simulink model "model_hippocampus"  (R2019b)
settings: Solver=ode23t  StartTime=0.0  StopTime=30  RelTol=1e-3
values from neighbouring files (symbols this model uses):
  C_T = 0.0000363    (= 3.63e-05)    [calculate_w_from_f_m.m]    (also in create_model-mummel-PC.m; create_model.m)
  D_l = -diag([X_u_u Y_v_v Z_w_w K_p_p M_q_q N_r_r])    [create_model-mummel-PC.m]    (also in create_model.m)
  D_r = -diag([X_u_u Y_v_v Z_w_w K_p_p M_q_q N_r_r])    [create_model-mummel-PC.m]    (also in create_model.m)
  F_to_xrpy = [1 1 1 1;k_m -k_m k_m -k_m ; -h/2 -h/2 h/2 h/2 ; h/2 -h/2 -h/2 h/2]    [calculate_w_from_f_m.m]    (also in create_model-mummel-PC.m = [1 1 1 1;-k_m k_m -k_m k_m ; -h/2 -h/2 h/2 h/2 ; h/2 -h/2 -h; create_model.m = [1 1 1 1;-k_m k_m -k_m k_m ; -h/2 -h/2 h/2 h/2 ; h/2 -h/2 -h)
  K = zeros(4,8)    [create_model-mummel-PC.m]    (also in create_model.m)
  K_list = [0.128176187695 -9.36648609631e-17 -5.00574293925e-18 -3.63491573314e-18 6.34309710249e-16 0.643960726702 1.98403777758e-15 -1.22713415344e-15 -1.03838985673e-16 -1.23229867768e-16 0.996702799245 2.36443760318e-16 ... (16384 elements, 4x8x512)]    [K_list_lqr_1_to_1.mat]    (also in K_list_lqr_moment.mat = [0.215933633332 5.36387970648e-15 5.12418514573e-17 4.256952; K_list_states_to_motor_force.mat = [0.101981554229 0.101981554229 0.101981554229 0.101981554229; create_model-mummel-PC.m = zeros(4,8,N*N*N); create_model.m = zeros(4,8,N*N*N))
  m = 1.47    [create_model-mummel-PC.m]    (also in create_model.m)
  M_A_11 = M_A(1:3,1:3)    [create_model-mummel-PC.m]    (also in create_model.m)
  M_A_22 = M_A(4:6,4:6)    [create_model-mummel-PC.m]    (also in create_model.m)
  M_RB_22 = M_RB(4:6,4:6)    [create_model-mummel-PC.m]    (also in create_model.m)
  M_RB_M_A_INV = inv(M_RB+M_A)    [create_model-mummel-PC.m]    (also in create_model.m)
  mix_matrix_trpy_to_velocity_motor = [[1 1 1 1]' [-1 1 -1 1]' [-1 -1 1 1]' [1 -1 -1 1]']*0.4    [check_correct_index.m]    (also in create_model-mummel-PC.m = [[1 1 1 1]' [-1 1 -1 1]' [-1 -1 1 1]' [1 -1 -1 1]']; create_model.m = [[1 1 1 1]' [-1 1 -1 1]' [-1 -1 1 1]' [1 -1 -1 1]'])
undefined symbols (not defined in the file or in its folder): sigbuilder_block
settings Model: Creator=mummel  LastModifiedBy=tim
settings SolverCC: ZeroCrossAlgorithm=Adaptive
settings DebuggingCC: IgnoredZcDiagnostic=none

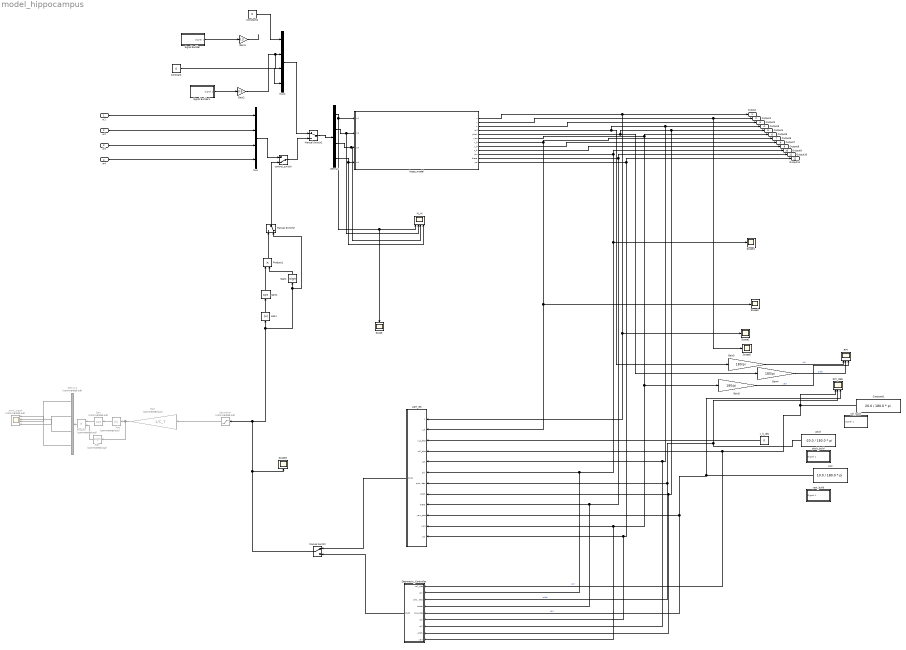
== system model_hippocampus ==
  w1 : Inport
  w2 : Inport  Port=2
  w3 : Inport  Port=3
  w4 : Inport  Port=4
  Abs : Abs  Commented=on
  Abs1 : Abs
  Constant : Constant  Value=0
  Constant1 : Constant  Value=20.0 / 180.0 * pi
  Constant2 : Constant  Value=0
  Demux : Demux
  Demux1 : Demux  Commented=on
  Gain : Gain  Commented=on  Gain=1/C_T
  Gain1 : Gain  Gain=0.3
  Gain2 : Gain  Gain=0.6
  Gain3 : Gain  Gain=180/pi
  Gain4 : Gain  Gain=180/pi
  Gain5 : Gain  Gain=180/pi
  Geometric_Controller : Subsystem
  LQR_GS : Subsystem
  M_IN : Scope  NumInputPorts=4
  Manual Switch : ManualSwitch
  Manual Switch1 : ManualSwitch
  Manual Switch2 : ManualSwitch  CurrentSetting=0
  Mux : Mux
  Mux2 : Mux
  Product : Product  Commented=on
  Product1 : Product
  RPY : Scope  NumInputPorts=3
  RPY_DES : Scope  NumInputPorts=3
  Saturation : Saturate  Commented=on  UpperLimit=7  LowerLimit=-7
  Scope{,1..5} (6 alike) : Scope
  Sign : Signum  Commented=on
  Sign1 : Signum
  Signal Builder : Subsystem  Tag=STV Subsys  LoadFcn=sigbuilder_block('load');  StartFcn=sigbuilder_block('start');  StopFcn=sigbuilder_block('stop');  ClipboardFcn=sigbuilder_block('clipboard');  mask(Sigbuilder block){tuvar=[0:10]}
      mask help: Simulink:masks:SigbuilderBlock_MD
      mask init:
      | if ~strcmp(get_param(bdroot(gcbh),'SimulationStatus'),'stopped') tuvar = sigbuilder_block('maskInit'); end
      settings: CopyFcn=sigbuilder_block('copy');  DeleteFcn=sigbuilder_block('delete');  ModelCloseFcn=sigbuilder_block('modelClose');  PreSaveFcn=sigbuilder_block('preSave');  PauseFcn=sigbuilder_block('pause');  ContinueFcn=sigbuilder_block('continue');  NameChangeFcn=sigbuilder_block('namechange');  OpenFcn=sigbuilder_block('open',[864 302.4 573.726 359.242 ]);  CloseFcn=sigbuilder_block('close');
      mask Display: plot(0, 0, 100, 100,[2, 2, 32, 32, 2], [68, 8, 8, 68, 68],[32, 2], [38, 38], [32, 19, 2],[53, 60, 44], [32, 17, 17, 2],[16, 16, 31, 31]);txt = getActiveGroup(gcbh);text(2, 100, txt,'verticalAlignment', 'top');
  Signal Builder1 : Subsystem  Tag=STV Subsys  LoadFcn=sigbuilder_block('load');  StartFcn=sigbuilder_block('start');  StopFcn=sigbuilder_block('stop');  ClipboardFcn=sigbuilder_block('clipboard');  mask(Sigbuilder block){tuvar=[0:10]}
      mask help: Simulink:masks:SigbuilderBlock_MD
      mask init:
      | if ~strcmp(get_param(bdroot(gcbh),'SimulationStatus'),'stopped') tuvar = sigbuilder_block('maskInit'); end
      settings: CopyFcn=sigbuilder_block('copy');  DeleteFcn=sigbuilder_block('delete');  ModelCloseFcn=sigbuilder_block('modelClose');  PreSaveFcn=sigbuilder_block('preSave');  PauseFcn=sigbuilder_block('pause');  ContinueFcn=sigbuilder_block('continue');  NameChangeFcn=sigbuilder_block('namechange');  OpenFcn=sigbuilder_block('open',[780.75 95.25 558.75 317.25 ]);  CloseFcn=sigbuilder_block('close');
      mask Display: plot(0, 0, 100, 100,[2, 2, 32, 32, 2], [68, 8, 8, 68, 68],[32, 2], [38, 38], [32, 19, 2],[53, 60, 44], [32, 17, 17, 2],[16, 16, 31, 31]);txt = getActiveGroup(gcbh);text(2, 100, txt,'verticalAlignment', 'top');
  Sqrt : Sqrt  Commented=on  SaturateOnIntegerOverflow=on
  Sqrt1 : Sqrt  SaturateOnIntegerOverflow=on
  control_switch : ManualSwitch  CurrentSetting=0
  hippo_model : Subsystem
  pitch : Constant  Value=-20.0 / 180.0 * pi
  pitch_build : Subsystem  Tag=STV Subsys  LoadFcn=sigbuilder_block('load');  StartFcn=sigbuilder_block('start');  StopFcn=sigbuilder_block('stop');  ClipboardFcn=sigbuilder_block('clipboard');  mask(Sigbuilder block){tuvar=[0:10]}
      mask help: Simulink:masks:SigbuilderBlock_MD
      mask init:
      | if ~strcmp(get_param(bdroot(gcbh),'SimulationStatus'),'stopped') tuvar = sigbuilder_block('maskInit'); end
      settings: CopyFcn=sigbuilder_block('copy');  DeleteFcn=sigbuilder_block('delete');  ModelCloseFcn=sigbuilder_block('modelClose');  PreSaveFcn=sigbuilder_block('preSave');  PauseFcn=sigbuilder_block('pause');  ContinueFcn=sigbuilder_block('continue');  NameChangeFcn=sigbuilder_block('namechange');  OpenFcn=sigbuilder_block('open',[437.6 199.2 550.4 400 ]);  CloseFcn=sigbuilder_block('close');
      mask Display: plot(0, 0, 100, 100,[2, 2, 32, 32, 2], [68, 8, 8, 68, 68],[32, 2], [38, 38], [32, 19, 2],[53, 60, 44], [32, 17, 17, 2],[16, 16, 31, 31]);txt = getActiveGroup(gcbh);text(2, 100, txt,'verticalAlignment', 'top');
  pwm_signal : Scope  Commented=on  NumInputPorts=4
  roll_build : Subsystem  Tag=STV Subsys  LoadFcn=sigbuilder_block('load');  StartFcn=sigbuilder_block('start');  StopFcn=sigbuilder_block('stop');  ClipboardFcn=sigbuilder_block('clipboard');  mask(Sigbuilder block){tuvar=[0:10]}
      mask help: Simulink:masks:SigbuilderBlock_MD
      mask init:
      | if ~strcmp(get_param(bdroot(gcbh),'SimulationStatus'),'stopped') tuvar = sigbuilder_block('maskInit'); end
      settings: CopyFcn=sigbuilder_block('copy');  DeleteFcn=sigbuilder_block('delete');  ModelCloseFcn=sigbuilder_block('modelClose');  PreSaveFcn=sigbuilder_block('preSave');  PauseFcn=sigbuilder_block('pause');  ContinueFcn=sigbuilder_block('continue');  NameChangeFcn=sigbuilder_block('namechange');  OpenFcn=sigbuilder_block('open',[437.6 199.2 550.4 400 ]);  CloseFcn=sigbuilder_block('close');
      mask Display: plot(0, 0, 100, 100,[2, 2, 32, 32, 2], [68, 8, 8, 68, 68],[32, 2], [38, 38], [32, 19, 2],[53, 60, 44], [32, 17, 17, 2],[16, 16, 31, 31]);txt = getActiveGroup(gcbh);text(2, 100, txt,'verticalAlignment', 'top');
  x_b_des : Constant  Value=0
  yaw : Constant  Value=10.0 / 180.0 * pi
  yaw_build : Subsystem  Tag=STV Subsys  LoadFcn=sigbuilder_block('load');  StartFcn=sigbuilder_block('start');  StopFcn=sigbuilder_block('stop');  ClipboardFcn=sigbuilder_block('clipboard');  mask(Sigbuilder block){tuvar=[0:10]}
      mask help: Simulink:masks:SigbuilderBlock_MD
      mask init:
      | if ~strcmp(get_param(bdroot(gcbh),'SimulationStatus'),'stopped') tuvar = sigbuilder_block('maskInit'); end
      settings: CopyFcn=sigbuilder_block('copy');  DeleteFcn=sigbuilder_block('delete');  ModelCloseFcn=sigbuilder_block('modelClose');  PreSaveFcn=sigbuilder_block('preSave');  PauseFcn=sigbuilder_block('pause');  ContinueFcn=sigbuilder_block('continue');  NameChangeFcn=sigbuilder_block('namechange');  OpenFcn=sigbuilder_block('open',[437.6 199.2 550.4 400 ]);  CloseFcn=sigbuilder_block('close');
      mask Display: plot(0, 0, 100, 100,[2, 2, 32, 32, 2], [68, 8, 8, 68, 68],[32, 2], [38, 38], [32, 19, 2],[53, 60, 44], [32, 17, 17, 2],[16, 16, 31, 31]);txt = getActiveGroup(gcbh);text(2, 100, txt,'verticalAlignment', 'top');
  Output : Outport
  Output1 : Outport  Port=2
  Output2 : Outport  Port=3
  Output3 : Outport  Port=4
  Output4 : Outport  Port=5
  Output5 : Outport  Port=6
  Output6 : Outport  Port=7
  Output7 : Outport  Port=8
  Output8 : Outport  Port=9
  Output9 : Outport  Port=10
  Output10 : Outport  Port=11
  Output11 : Outport  Port=12
  wires:
  w4/1 -> Mux/4
  w3/1 -> Mux/3
  w2/1 -> Mux/2
  w1/1 -> Mux/1
  hippo_model/1(x) -> Output/1, LQR_GS/1(x), Scope1/1
  hippo_model/2(y) -> Scope5/1, Output1/1
  hippo_model/3(z) -> Output2/1
  hippo_model/4(roll) -> Geometric_Controller/7(roll), LQR_GS/5(roll), Output3/1, Gain3/1
  hippo_model/5(pitch) -> Geometric_Controller/8(pitch), LQR_GS/8(pitch), Output4/1, Gain4/1
  hippo_model/6(yaw) -> Gain5/1, Geometric_Controller/9(yaw), LQR_GS/11(yaw), Output5/1
  hippo_model/7(x_b) -> Output6/1, Scope2/1, LQR_GS/2(x_b)
  hippo_model/8(y_b) -> Output7/1
  hippo_model/9(z_b) -> Output8/1
  hippo_model/10(phi) -> Output9/1, Geometric_Controller/2(phi), LQR_GS/6(phi), Scope4/1
  hippo_model/11(theta) -> Output10/1, LQR_GS/9(theta), Geometric_Controller/4(theta)
  hippo_model/12(psi) -> Output11/1, Geometric_Controller/6(psi), LQR_GS/12(psi)
  Mux/1 -> control_switch/1
  control_switch/1 -> Manual Switch1/2
  Manual Switch/1 -> Scope3/1, Manual Switch2/2, Sign1/1, Abs1/1, Saturation/1
  yaw/1 -> Geometric_Controller/5(yaw_des), LQR_GS/10(yaw_des), RPY_DES/3  "yaw"
  Mux2/1 -> Manual Switch1/1
  Manual Switch1/1 -> Demux/1
  Demux/1 -> hippo_model/1(w1), Scope/1, M_IN/1
  Demux/2 -> hippo_model/2(w2), M_IN/2
  Demux/3 -> hippo_model/3(w3), M_IN/3
  Demux/4 -> hippo_model/4(w4), M_IN/4
  Signal Builder/1(Signal 1) -> Gain1/1
  Geometric_Controller/1(Out1) -> Manual Switch/2
  x_b_des/1 -> LQR_GS/3(x_b_des)
  LQR_GS/1(Out1) -> Manual Switch/1
  Abs/1 -> Sqrt/1
  Sqrt/1 -> Product/1
  Demux1/4 -> pwm_signal/1
  Demux1/3 -> pwm_signal/2
  Demux1/2 -> pwm_signal/4
  Demux1/1 -> pwm_signal/3
  Saturation/1 -> Gain/1
  Gain/1 -> Sign/1, Abs/1
  Sign/1 -> Product/2
  Product/1 -> Demux1/1
  Signal Builder1/1(Signal 1) -> Gain2/1
  Constant1/1 -> RPY_DES/1, Geometric_Controller/1(roll_des), LQR_GS/4(roll_des)  "roll"
  pitch/1 -> Geometric_Controller/3(pitch_des), LQR_GS/7(pitch_des), RPY_DES/2  "pitch"
  Constant/1 -> Mux2/4
  Gain3/1 -> RPY/1  "roll"
  Gain5/1 -> RPY/3  "yaw"
  Gain4/1 -> RPY/2  "pitch"
  Manual Switch2/1 -> control_switch/2
  Abs1/1 -> Sqrt1/1
  Sign1/1 -> Product1/2
  Sqrt1/1 -> Product1/1
  Product1/1 -> Manual Switch2/1
  Gain2/1 -> Mux2/3, Mux2/2
  Gain1/1 -> ?
  Constant2/1 -> Mux2/1

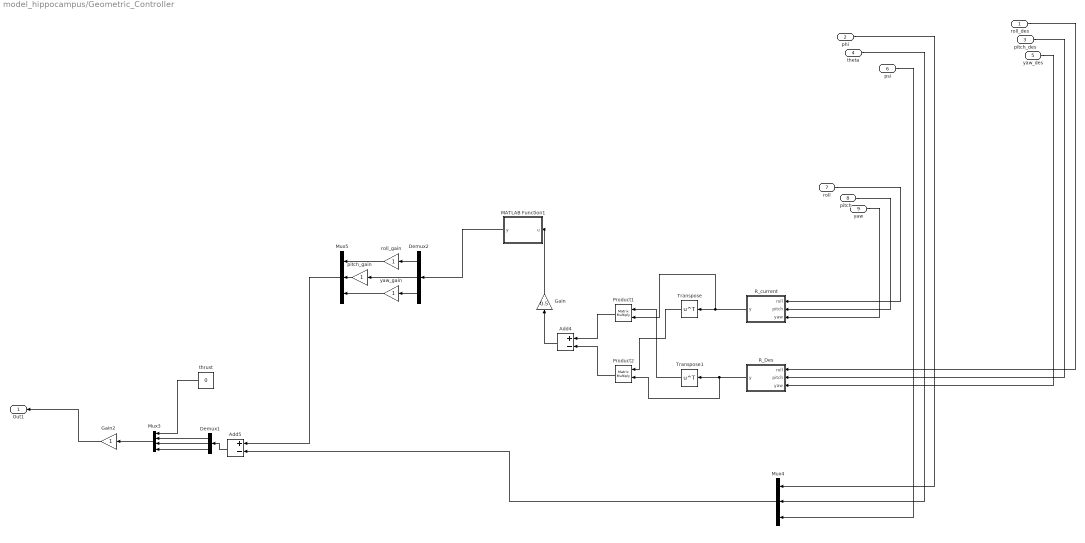
== system model_hippocampus/Geometric_Controller ==
  roll_des : Inport
  phi : Inport  Port=2
  pitch_des : Inport  Port=3
  theta : Inport  Port=4
  yaw_des : Inport  Port=5
  psi : Inport  Port=6
  roll : Inport  Port=7
  pitch : Inport  Port=8
  yaw : Inport  Port=9
  Add4 : Sum  Inputs=+-
  Add5 : Sum  Inputs=+-
  Demux1 : Demux  Outputs=3
  Demux2 : Demux  Outputs=3
  Gain : Gain  Gain=0.5
  Gain2 : Gain
  MATLAB Function1 : MATLAB Function  TreatAsAtomicUnit=on
  Mux3 : Mux
  Mux4 : Mux  Inputs=3
  Mux5 : Mux  Inputs=3
  Product1 : Product  Multiplication=Matrix(*)
  Product2 : Product  Multiplication=Matrix(*)
  R_Des : MATLAB Function  TreatAsAtomicUnit=on
  R_current : MATLAB Function  TreatAsAtomicUnit=on
  Transpose : Math  Operator=transpose  SignedPower=off  SaturateOnIntegerOverflow=on
  Transpose1 : Math  Operator=transpose  SignedPower=off  SaturateOnIntegerOverflow=on
  pitch_gain : Gain
  roll_gain : Gain
  thrust : Constant  Value=0
  yaw_gain : Gain
  Out1 : Outport
  wires:
  Transpose/1 -> Product2/1
  roll_des/1 -> R_Des/1(roll)
  Add5/1 -> Demux1/1
  roll_gain/1 -> Mux5/1
  Demux2/1 -> roll_gain/1
  phi/1 -> Mux4/1
  MATLAB Function1/1(y) -> Demux2/1
  Demux1/3 -> Mux3/4
  Demux1/2 -> Mux3/3
  psi/1 -> Mux4/3
  R_Des/1(y) -> Product2/2, Transpose1/1
  Product2/1 -> Add4/2
  Mux4/1 -> Add5/2
  R_current/1(y) -> Product1/2, Transpose/1
  Mux3/1 -> Gain2/1
  roll/1 -> R_current/1(roll)
  Demux2/2 -> pitch_gain/1
  yaw/1 -> R_current/3(yaw)
  Demux1/1 -> Mux3/2
  theta/1 -> Mux4/2
  pitch_gain/1 -> Mux5/2
  yaw_des/1 -> R_Des/3(yaw)
  pitch_des/1 -> R_Des/2(pitch)
  Demux2/3 -> yaw_gain/1
  yaw_gain/1 -> Mux5/3
  thrust/1 -> Mux3/1
  Gain/1 -> MATLAB Function1/1(u)
  Transpose1/1 -> Product1/1
  Product1/1 -> Add4/1
  Gain2/1 -> Out1/1
  Add4/1 -> Gain/1
  Mux5/1 -> Add5/1
  pitch/1 -> R_current/2(pitch)

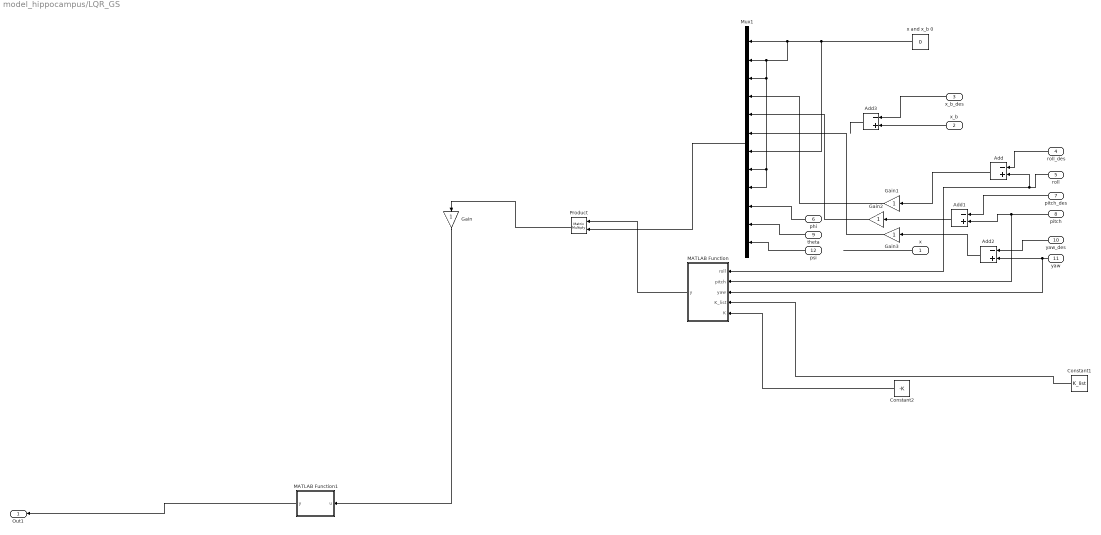
== system model_hippocampus/LQR_GS ==
  x : Inport
  x_b : Inport  Port=2
  x_b_des : Inport  Port=3
  roll_des : Inport  Port=4
  roll : Inport  Port=5
  phi : Inport  Port=6
  pitch_des : Inport  Port=7
  pitch : Inport  Port=8
  theta : Inport  Port=9
  yaw_des : Inport  Port=10
  yaw : Inport  Port=11
  psi : Inport  Port=12
  Add{,1..3} (4 alike) : Sum  Inputs=-+
  Constant1 : Constant  Value=K_list
  Constant2 : Constant  Value=-K
  Gain{,1..3} (4 alike) : Gain
  MATLAB Function : MATLAB Function  TreatAsAtomicUnit=on
  MATLAB Function1 : MATLAB Function  TreatAsAtomicUnit=on
  Mux1 : Mux  Inputs=12
  Product : Product  Multiplication=Matrix(*)
  x and x_b 0 : Constant  Value=0
  Out1 : Outport
  wires:
  Add/1 -> Gain1/1
  x_b_des/1 -> Add3/1
  MATLAB Function/1(y) -> Product/1
  yaw/1 -> Add2/2, MATLAB Function/3(yaw)
  Add1/1 -> Gain2/1
  Constant2/1 -> MATLAB Function/5(K)
  Add3/1 -> ?
  pitch_des/1 -> Add1/1
  Constant1/1 -> MATLAB Function/4(K_list)
  Gain/1 -> MATLAB Function1/1(u)
  Add2/1 -> Gain3/1
  pitch/1 -> Add1/2, MATLAB Function/2(pitch)
  Mux1/1 -> Product/2
  yaw_des/1 -> Add2/1
  x_b/1 -> Add3/2
  Product/1 -> Gain/1
  roll/1 -> Add/2, MATLAB Function/1(roll)
  roll_des/1 -> Add/1
  MATLAB Function1/1(y) -> Out1/1
  Gain1/1 -> Mux1/4
  Gain2/1 -> Mux1/5
  Gain3/1 -> Mux1/6
  x and x_b 0/1 -> Mux1/7, Mux1/9, Mux1/8, Mux1/3, Mux1/2, Mux1/1
  phi/1 -> Mux1/10
  theta/1 -> Mux1/11
  psi/1 -> Mux1/12
  x/1 -> ?

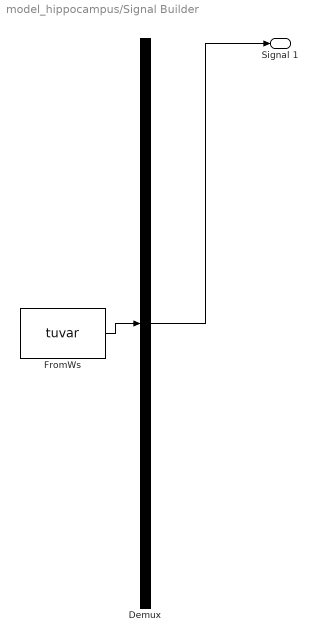
== system model_hippocampus/Signal Builder ==
  Demux : Demux  Tag=STV Demux  Outputs=1
  FromWs : FromWorkspace  Tag=STV FromWs  VariableName=tuvar  SampleTime=0
      SigBuilderData=|
      | common.afterFinalStr = 'Extrapolate'
      | common.sampleTime = 0
      | dataSet.timeRange = [0 10]
      | dataSet.name = 'Group 1'
      | sbobj.Groups.Name = 'Group 1'
      | sbobj.Groups.Signals.Name = 'Signal 1'
      | sbobj.Groups.Signals.XData = [0 2 2 8.04 8.04 10]
      | sbobj.Groups.Signals.YData = [0 0 0.59 0.59 0 0]
  Signal 1 : Outport  Tag=STV Outport
  wires:
  Demux/1 -> Signal 1/1
  FromWs/1 -> Demux/1

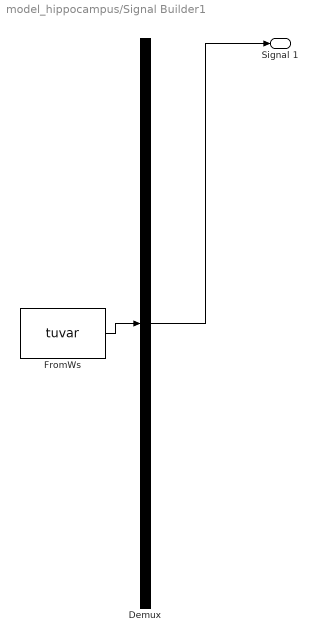
== system model_hippocampus/Signal Builder1 ==
  Demux : Demux  Tag=STV Demux  Outputs=1
  FromWs : FromWorkspace  Tag=STV FromWs  VariableName=tuvar  SampleTime=0
      SigBuilderData=|
      | common.afterFinalStr = 'Extrapolate'
      | common.sampleTime = 0
      | dataSet.timeRange = [0 10]
      | dataSet.name = 'Group 1'
      | sbobj.Groups.Name = 'Group 1'
      | sbobj.Groups.Signals.Name = 'Signal 1'
      | sbobj.Groups.Signals.XData = [0 4.98 4.98 5.98 5.98 10]
      | sbobj.Groups.Signals.YData = [0 0 0.89 0.89 0 0]
  Signal 1 : Outport  Tag=STV Outport
  wires:
  Demux/1 -> Signal 1/1
  FromWs/1 -> Demux/1

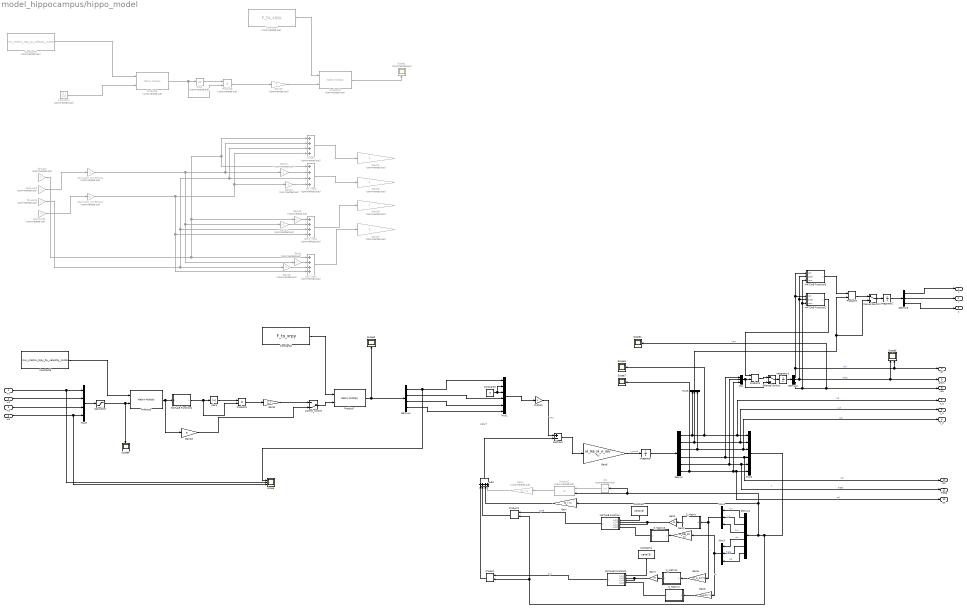
== system model_hippocampus/hippo_model ==
  note: INPUT
  note: v
  w1 : Inport
  w2 : Inport  Port=2
  w3 : Inport  Port=3
  w4 : Inport  Port=4
  Abs : Abs  Commented=on
  Abs1 : Abs
  Abs2 : Abs  Commented=on
  Add : Sum  Inputs=++++
  Constant : Constant  Value=zeros(3)
  Constant1 : Constant  Value=zeros(3)
  Constant2 : Constant  Value=0
  Constant3 : Constant  Value=F_to_xrpy
  Constant4 : Constant  Commented=on  Value=F_to_xrpy
  Constant5 : Constant  Value=mix_matrix_trpy_to_velocity_motor
  Constant6 : Constant  Commented=on  Value=mix_matrix_trpy_to_velocity_motor
  Constant7 : Constant  Commented=on  Value=[1 1 1 1]'
  Demux : Demux  Outputs=6
  Demux1 : Demux  Outputs=6
  Demux2 : Demux  Outputs=3
  Demux3 : Demux  Outputs=3
  Demux4 : Demux
  Gain : Gain  Gain=D_l  Multiplication=Matrix(K*u)
  Gain1 : Gain  Gain=-m
  Gain{9..14} (6 alike) : Gain  Commented=on  Gain=-1
  Gain15 : Gain  Commented=on  Gain=7
  Gain16 : Gain  Gain=9
  Gain{18..21} (4 alike) : Gain  Commented=on
  Gain2 : Gain  Gain=M_RB_22  Multiplication=Matrix(K*u)
  Gain3 : Gain  Gain=M_A_22  Multiplication=Matrix(K*u)
  Gain4 : Gain  Commented=on  Gain=D_r  Multiplication=Matrix(K*u)
  Gain5 : Gain  Gain=M_A_11  Multiplication=Matrix(K*u)
  Gain6 : Gain  Gain=M_RB_M_A_INV  Multiplication=Matrix(K*u)
  Gain7 : Gain  Gain=-m
  Gain8 : Gain  Gain=C_T
  Integrator : Integrator  ContinuousStateAttributes={'x_b', 'y_b', 'z_b','phi', 'theta', 'psi'}
  Integrator1 : Integrator  InitialCondition=[0 0 0]  ContinuousStateAttributes={'roll', 'pitch', 'yaw'}
  Integrator2 : Integrator  ContinuousStateAttributes={'x', 'y', 'z'}
  MATLAB Function : MATLAB Function  TreatAsAtomicUnit=on
  MATLAB Function1 : MATLAB Function  TreatAsAtomicUnit=on
  MATLAB Function2 : MATLAB Function  TreatAsAtomicUnit=on
  MATLAB Function3 : MATLAB Function  TreatAsAtomicUnit=on
  MATLAB Function4 : MATLAB Function  TreatAsAtomicUnit=on
  Manual Switch : ManualSwitch
  Manual Switch1 : ManualSwitch
  Multiply : Gain
  Mux{,3..5} (4 alike) : Mux  Inputs=3
  Mux1 : Mux  Inputs=6
  Mux2 : Mux  Inputs=6
  Mux6 : Mux
  Product{,1,3..4,6..7} (6 alike) : Product  Multiplication=Matrix(*)
  Product10 : Product  Commented=on  Multiplication=Matrix(*)
  Product2 : Product  Commented=on
  Product5 : Product
  Product8 : Product  Commented=on
  Product9 : Product  Commented=on  Multiplication=Matrix(*)
  S_Matrix : MATLAB Function  TreatAsAtomicUnit=on
  S_Matrix1 : MATLAB Function  TreatAsAtomicUnit=on
  S_Matrix2 : MATLAB Function  TreatAsAtomicUnit=on
  S_Matrix3 : MATLAB Function  TreatAsAtomicUnit=on
  Saturation : Saturate
  Scope : Scope  NumInputPorts=3
  Scope1 : Scope  Commented=on
  Scope{2..4,6..7} (5 alike) : Scope
  Scope5 : Scope  NumInputPorts=2
  Subtract : Sum  Inputs=+-
  backward : Gain  Commented=on  Gain=-1
  backward1 : Gain  Commented=on  Gain=-1
  backward_correction1 : Gain  Commented=on  Gain=-1
  backward_correction2 : Gain  Commented=on  Gain=-1
  control_switch : ManualSwitch  CurrentSetting=0
  forward : Gain  Commented=on
  forward1 : Gain  Commented=on
  pitch_input : Sum  Commented=on  Inputs=++++
  roll_input : Sum  Commented=on  Inputs=++++
  thrust : Sum  Commented=on  Inputs=++++
  yaw_input : Sum  Commented=on  Inputs=++++
  x : Outport
  y : Outport  Port=2
  z : Outport  Port=3
  roll : Outport  Port=4
  pitch : Outport  Port=5
  yaw : Outport  Port=6
  x_b : Outport  Port=7
  y_b : Outport  Port=8
  z_b : Outport  Port=9
  phi : Outport  Port=10
  theta : Outport  Port=11
  psi : Outport  Port=12
  wires:
  Demux/6 -> Scope7/1, Mux/3, psi/1, Mux2/6  "psi"
  S_Matrix3/1(y) -> MATLAB Function/4(u_22)
  Demux/5 -> Mux/2, theta/1, Mux2/5  "theta"
  Gain1/1 -> MATLAB Function/3(u_21), MATLAB Function/2(u_12)
  Mux1/1 -> Multiply/1
  Gain6/1 -> Integrator/1  "V_punkt"
  MATLAB Function1/1(y) -> Product/1  "C_A"
  Demux2/3 -> Scope4/1, yaw/1, MATLAB Function3/3(yaw), MATLAB Function2/3(yaw)  "yaw"
  Demux/2 -> y_b/1, Mux2/2, Mux5/2  "y_b"
  Demux2/2 -> Scope5/1, pitch/1, MATLAB Function2/2(pitch), MATLAB Function3/2(pitch)  "pitch"
  Demux/4 -> Mux/1, phi/1, Mux2/4  "phi"
  Integrator1/1 -> Demux2/1
  MATLAB Function/1(y) -> Product1/1  "C_RB"
  S_Matrix/1(y) -> Gain1/1
  Product1/1 -> Add/2
  Constant1/1 -> MATLAB Function1/1(u_11)
  Gain7/1 -> MATLAB Function1/2(u_12), MATLAB Function1/3(u_21)
  Gain/1 -> Add/3
  Demux2/1 -> MATLAB Function2/1(roll), MATLAB Function3/1(roll), Scope5/2, roll/1  "roll"
  Demux/3 -> z_b/1, Mux2/3, Mux5/3  "z_b"
  Add/1 -> Subtract/2
  Product/1 -> Add/1
  Demux/1 -> Scope3/1, x_b/1, Mux2/1, Mux5/1  "x_b"
  Mux2/1 -> Product/2, Product1/2, Abs/1, Product2/2, Gain/1, Demux1/1
  Constant2/1 -> Mux1/2, Mux1/3
  Product2/1 -> Gain4/1
  Demux1/5 -> Mux3/2  "theta"
  Mux3/1 -> Gain3/1, Gain2/1  "w"
  Gain4/1 -> Add/4
  S_Matrix1/1(y) -> MATLAB Function1/4(u_22)
  Gain3/1 -> S_Matrix1/1(u)
  Integrator/1 -> Demux/1
  Multiply/1 -> Subtract/1  "TAU"
  S_Matrix2/1(y) -> Gain7/1
  Demux1/3 -> Mux4/3  "z_w"
  Demux1/4 -> Mux3/1  "phi"
  Demux1/6 -> Mux3/3  "psi"
  Subtract/1 -> Gain6/1
  Product3/1 -> Manual Switch1/1
  Mux4/1 -> S_Matrix/1(u), Gain5/1  "v"
  Abs/1 -> Product2/1
  Gain2/1 -> S_Matrix3/1(u)
  Mux5/1 -> Manual Switch1/2, Product3/2
  MATLAB Function2/1(y) -> Product4/1
  Gain5/1 -> S_Matrix2/1(u)
  Demux3/2 -> y/1
  Demux1/1 -> Mux4/1  "x_w"
  Constant/1 -> MATLAB Function/1(u_11)
  Demux1/2 -> Mux4/2  "y_w"
  Demux3/1 -> x/1
  Demux3/3 -> z/1
  thrust/1 -> Gain21/1
  forward/1 -> roll_input/1, thrust/1, Gain13/1, yaw_input/1
  backward/1 -> backward_correction2/1
  forward1/1 -> roll_input/3, thrust/3, pitch_input/3, Gain10/1
  backward1/1 -> backward_correction1/1
  backward_correction2/1 -> Gain9/1, Gain14/1, Gain11/1, thrust/2
  backward_correction1/1 -> thrust/4, Gain12/1, yaw_input/4, pitch_input/4
  roll_input/1 -> Gain18/1
  Gain9/1 -> yaw_input/2
  Gain10/1 -> yaw_input/3
  Gain12/1 -> roll_input/4
  Gain11/1 -> roll_input/2
  yaw_input/1 -> Gain20/1
  Gain14/1 -> pitch_input/2
  Gain13/1 -> pitch_input/1
  pitch_input/1 -> Gain19/1
  Integrator2/1 -> Demux3/1
  Manual Switch/1 -> Integrator1/1
  Mux/1 -> Manual Switch/2, Product4/2
  Product4/1 -> Manual Switch/1
  Manual Switch1/1 -> Integrator2/1
  Demux4/1 -> Scope/1, Mux1/1
  Demux4/2 -> Mux1/4
  Demux4/4 -> Mux1/6
  Demux4/3 -> Mux1/5
  Constant3/1 -> Product7/1
  MATLAB Function4/1(y) -> Abs1/1, Product5/2
  Constant5/1 -> Product6/1
  Abs1/1 -> Product5/1
  Mux6/1 -> Saturation/1
  Product7/1 -> Demux4/1, Scope2/1
  Constant4/1 -> Product10/1
  Constant7/1 -> Product9/2
  Product8/1 -> Gain15/1
  Constant6/1 -> Product9/1
  Abs2/1 -> Product8/1
  Gain15/1 -> Product10/2
  Product9/1 -> Product8/2, Abs2/1
  Product10/1 -> Scope1/1
  Product5/1 -> Gain8/1
  Product6/1 -> Gain16/1, MATLAB Function4/1(p)
  Gain16/1 -> control_switch/2
  control_switch/1 -> Product7/2
  Gain8/1 -> control_switch/1
  MATLAB Function3/1(y) -> Product3/1
  w1/1 -> Scope/2, Mux6/1
  w2/1 -> Mux6/2
  w3/1 -> Mux6/3
  w4/1 -> Scope/3, Mux6/4
  Saturation/1 -> Scope6/1, Product6/2

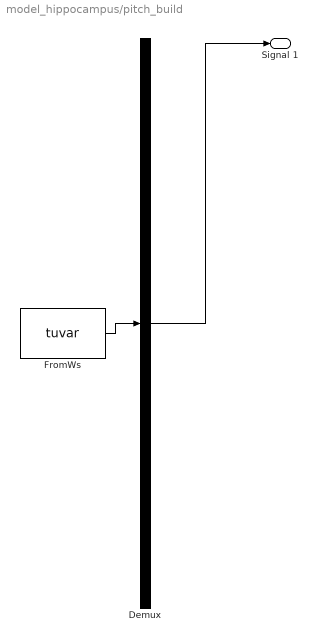
== system model_hippocampus/pitch_build ==
  Demux : Demux  Tag=STV Demux  Outputs=1
  FromWs : FromWorkspace  Tag=STV FromWs  VariableName=tuvar  SampleTime=0
      SigBuilderData=|
      | common.afterFinalStr = 'Extrapolate'
      | common.sampleTime = 0
      | dataSet.timeRange = [0 10]
      | dataSet.name = 'Group 1'
      | sbobj.Groups.Name = 'Group 1'
      | sbobj.Groups.Signals.Name = 'Signal 1'
      | sbobj.Groups.Signals.XData = [0 1 1 6 6 10]
      | sbobj.Groups.Signals.YData = [0 0 1 1 0 0]
  Signal 1 : Outport  Tag=STV Outport
  wires:
  Demux/1 -> Signal 1/1
  FromWs/1 -> Demux/1

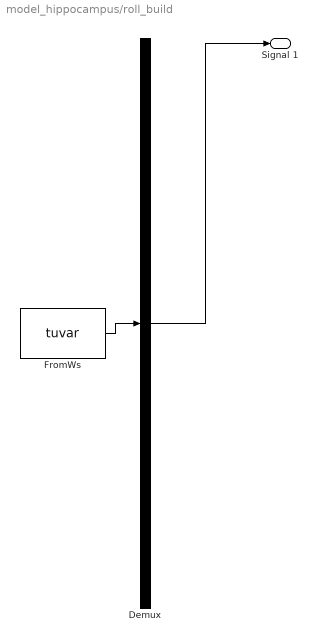
== system model_hippocampus/roll_build ==
  Demux : Demux  Tag=STV Demux  Outputs=1
  FromWs : FromWorkspace  Tag=STV FromWs  VariableName=tuvar  SampleTime=0
      SigBuilderData=|
      | common.afterFinalStr = 'Extrapolate'
      | common.sampleTime = 0
      | dataSet.timeRange = [0 10]
      | dataSet.name = 'Group 1'
      | sbobj.Groups.Name = 'Group 1'
      | sbobj.Groups.Signals.Name = 'Signal 1'
      | sbobj.Groups.Signals.XData = [0 1.02 1.02 3 3 10]
      | sbobj.Groups.Signals.YData = [0 0 1 0.595 0 0]
  Signal 1 : Outport  Tag=STV Outport
  wires:
  Demux/1 -> Signal 1/1
  FromWs/1 -> Demux/1

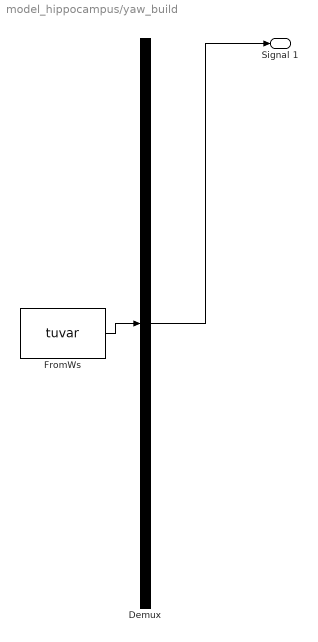
== system model_hippocampus/yaw_build ==
  Demux : Demux  Tag=STV Demux  Outputs=1
  FromWs : FromWorkspace  Tag=STV FromWs  VariableName=tuvar  SampleTime=0
      SigBuilderData=|
      | common.afterFinalStr = 'Extrapolate'
      | common.sampleTime = 0
      | dataSet.timeRange = [0 10]
      | dataSet.name = 'Group 1'
      | sbobj.Groups.Name = 'Group 1'
      | sbobj.Groups.Signals.Name = 'Signal 1'
      | sbobj.Groups.Signals.XData = [0 1.98 1.98 6 6 10]
      | sbobj.Groups.Signals.YData = [0 0 0.205 -0.755 0 0]
  Signal 1 : Outport  Tag=STV Outport
  wires:
  Demux/1 -> Signal 1/1
  FromWs/1 -> Demux/1

== matlab function model_hippocampus/hippo_model/MATLAB Function1 ==
  data: u_11 input; y output; u_12 input; u_21 input; u_22 input
function y = fcn(u_11,u_12,u_21,u_22)

y = [u_11 u_12; u_21 u_22];

== matlab function model_hippocampus/hippo_model/MATLAB Function ==
  data: u_11 input; y output; u_12 input; u_21 input; u_22 input
function y = fcn(u_11,u_12,u_21,u_22)

y = [u_11 u_12; u_21 u_22];

== matlab function model_hippocampus/hippo_model/S_Matrix ==
  data: u input size=3; y output
function y = fcn(u)

y = cross(repmat(u,1,3),eye(3,3)) ;

== matlab function model_hippocampus/hippo_model/S_Matrix1 ==
  data: u input; y output
function y = fcn(u)

y = cross(repmat(u,1,3),eye(3,3)) ;

== matlab function model_hippocampus/hippo_model/S_Matrix2 ==
  data: u input; y output
function y = fcn(u)
y = cross(repmat(u,1,3),eye(3,3)) ;

== matlab function model_hippocampus/hippo_model/S_Matrix3 ==
  data: u input size=3; y output
function y = fcn(u)

y = cross(repmat(u,1,3),eye(3,3)) ;

== matlab function model_hippocampus/hippo_model/MATLAB Function2 ==
  data: roll input; y output; pitch input; yaw input
function y = fcn(roll,pitch,yaw)
alpha = yaw
beta = pitch
gamma = roll
R_roll=[1 0 +sin(pitch);0 cos(roll) -sin(roll)+sin(pitch);0 sin(roll) cos(roll)]
%R_roll=[1 0 0;0 cos(roll) -sin(roll);0 sin(roll) cos(roll)]
% R_pitch=[cos(pitch) 0 sin(pitch);0 1 0; -sin(pitch) 0 cos(pitch)]
% R_yaw=[cos(yaw) -sin(yaw) 0; sin(yaw) cos(yaw) 0; 0 0 1]



R=[cos(alpha)*cos(beta) cos(alpha)*sin(beta)*sin(gamma)-sin(alpha)*cos(gamma) cos(alpha)*sin(beta)*cos(gamma)+sin(alpha)*sin(gamma);
  sin(alpha)*cos(beta) sin(alpha)*sin(beta)*sin(gamma)+cos(alpha)*cos(gamma) sin(alpha)*sin(beta)*cos(gamma)-cos(alpha)*sin(gamma);
  -sin(beta) cos(beta)*sin(gamma) cos(beta)*cos(gamma)];
y = R_roll

== matlab function model_hippocampus/LQR_GS/MATLAB Function ==
  data: roll input; y output; pitch input; yaw input; K_list input; K input
function y = fcn(roll,pitch,yaw,K_list,K)
N=16;
roll_list = linspace(0,2*pi,N);
pitch_list = linspace(0,2*pi,N);
yaw_list = linspace(0,2*pi,N);

[M,index_roll]=min(abs(roll_list-roll));
[M,index_pitch]=min(abs(pitch_list-pitch));
[M,index_yaw]=min(abs(yaw_list-yaw));
index=(index_roll-1)*N*N+(index_pitch-1)*N+index_yaw
%yaw_index = (yaw_body/(2.0*3.14159/(7.0)));
%pitch_index = (pitch_body/(2.0*3.14159/(7.0)));
%roll_index = (roll_body/(2.0*3.14159/(7.0)));
%index=(roll_index)*64+(pitch_index)*8+yaw_index;
p=-1*K_list(:,:,index);
%p=-K_list(:,:,1);
y = p;

== matlab function model_hippocampus/Geometric_Controller/R_Des ==
  data: roll input; y output; pitch input; yaw input
function y = fcn(roll,pitch,yaw)
alpha = yaw
beta = pitch
gamma = roll
R=[cos(alpha)*cos(beta) cos(alpha)*sin(beta)*sin(gamma)-sin(alpha)*cos(gamma) cos(alpha)*sin(beta)*cos(gamma)+sin(alpha)*sin(gamma);
   sin(alpha)*cos(beta) sin(alpha)*sin(beta)*sin(gamma)+cos(alpha)*cos(gamma) sin(alpha)*sin(beta)*cos(gamma)-cos(alpha)*sin(gamma);
   -sin(beta) cos(beta)*sin(gamma) cos(beta)*cos(gamma)];
y = R

== matlab function model_hippocampus/Geometric_Controller/R_current ==
  data: roll input; y output; pitch input; yaw input
function y = fcn(roll,pitch,yaw)
alpha = yaw
beta = pitch
gamma = roll
R=[cos(alpha)*cos(beta) cos(alpha)*sin(beta)*sin(gamma)-sin(alpha)*cos(gamma) cos(alpha)*sin(beta)*cos(gamma)+sin(alpha)*sin(gamma);
   sin(alpha)*cos(beta) sin(alpha)*sin(beta)*sin(gamma)+cos(alpha)*cos(gamma) sin(alpha)*sin(beta)*cos(gamma)-cos(alpha)*sin(gamma);
   -sin(beta) cos(beta)*sin(gamma) cos(beta)*cos(gamma)];
y = R

== matlab function model_hippocampus/Geometric_Controller/MATLAB Function1 ==
  data: u input; y output
function y = fcn(u)

y = -[u(3,2) u(1,3) u(2,1)]';

== matlab function model_hippocampus/hippo_model/MATLAB Function3 ==
  data: roll input; y output; pitch input; yaw input
function y = fcn(roll,pitch,yaw)
alpha = yaw
beta = pitch
gamma = roll
R_roll=[1 0 +sin(pitch);0 cos(roll) -sin(roll)+sin(pitch);0 sin(roll) cos(roll)]
%R_roll=[1 0 0;0 cos(roll) -sin(roll);0 sin(roll) cos(roll)]
% R_pitch=[cos(pitch) 0 sin(pitch);0 1 0; -sin(pitch) 0 cos(pitch)]
% R_yaw=[cos(yaw) -sin(yaw) 0; sin(yaw) cos(yaw) 0; 0 0 1]



R=[cos(alpha)*cos(beta) cos(alpha)*sin(beta)*sin(gamma)-sin(alpha)*cos(gamma) cos(alpha)*sin(beta)*cos(gamma)+sin(alpha)*sin(gamma);
  sin(alpha)*cos(beta) sin(alpha)*sin(beta)*sin(gamma)+cos(alpha)*cos(gamma) sin(alpha)*sin(beta)*cos(gamma)-cos(alpha)*sin(gamma);
  -sin(beta) cos(beta)*sin(gamma) cos(beta)*cos(gamma)];
y = R

== matlab function model_hippocampus/hippo_model/MATLAB Function4 ==
  data: p input; y output
function y = fcn(p)

u=[0 0 0 0]'


u(1)=p(1)
u(2)=p(2)
u(3)=p(3)
u(4)=p(4)
for i=1:4
    if(u(i)>1)
        u(i)=1
    end
    if(u(i)<-1)
        u(i)=-1
    end
end

u=500*u


%if max(abs(u))>500
%    u=u/max(abs(u))*500
%end
y = u;

== matlab function model_hippocampus/LQR_GS/MATLAB Function1 ==
  data: u input; y output
function y = fcn(u)
y =[u(1,:);u(4,:);u(5,:);u(6,:)];
